simulink model "WaterTreatmentProcess"  (R2015b)
settings: Solver=VariableStepAuto  StartTime=0.0  StopTime=10.0  RelTol=1e-3
model workspace (MAT data in the model file):
  C0 = 1
  g = 9.81
  height = 1
  lenght = 12
  width = 3
settings Model: Creator=aemili  LastModifiedBy=andrea.emili

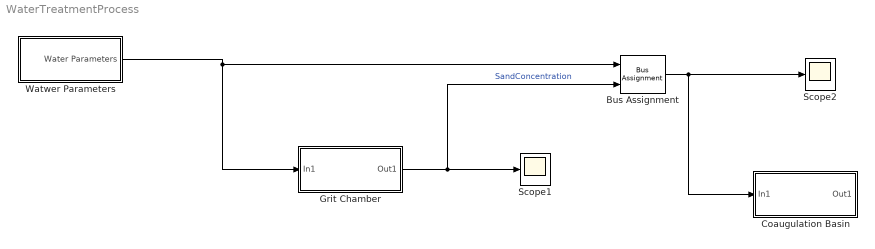
== system WaterTreatmentProcess ==
  Bus Assignment : BusAssignment  AssignedSignals=SandConcentration
  Coaugulation Basin : Subsystem
  Grit Chamber : Subsystem
  Scope1 : Scope
  Scope2 : Scope
  Watwer Parameters : Subsystem
  wires:
  Watwer Parameters/1(Water Parameters) -> Bus Assignment/1, Grit Chamber/1(In1)
  Grit Chamber/1(Out1) -> Bus Assignment/2, Scope1/1  "SandConcentration"
  Bus Assignment/1 -> Coaugulation Basin/1(In1), Scope2/1

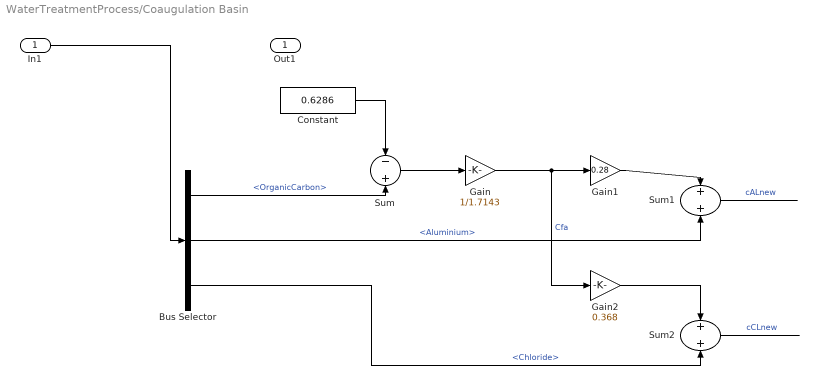
== system WaterTreatmentProcess/Coaugulation Basin ==
  In1 : Inport
  Bus Selector : BusSelector  OutputSignals=OrganicCarbon,Aluminium,Chloride
  Constant : Constant  Value=0.6286
  Gain : Gain  Gain=1/1.7143
  Gain1 : Gain  Gain=0.28
  Gain2 : Gain  Gain=0.368
  Sum : Sum  Inputs=-|+
  Sum1 : Sum  Inputs=+|+
  Sum2 : Sum  Inputs=+|+
  Out1 : Outport
  wires:
  In1/1 -> Bus Selector/1
  Sum/1 -> Gain/1
  Gain/1 -> Gain2/1, Gain1/1  "Cfa"
  Bus Selector/2 -> Sum1/2  "<Aluminium>"
  Bus Selector/3 -> Sum2/2  "<Chloride>"
  Gain1/1 -> Sum1/1
  Bus Selector/1 -> Sum/2  "<OrganicCarbon>"
  Constant/1 -> Sum/1
  Gain2/1 -> Sum2/1
  Sum2/1 -> ?  "cCLnew"
  Sum1/1 -> ?  "cALnew"

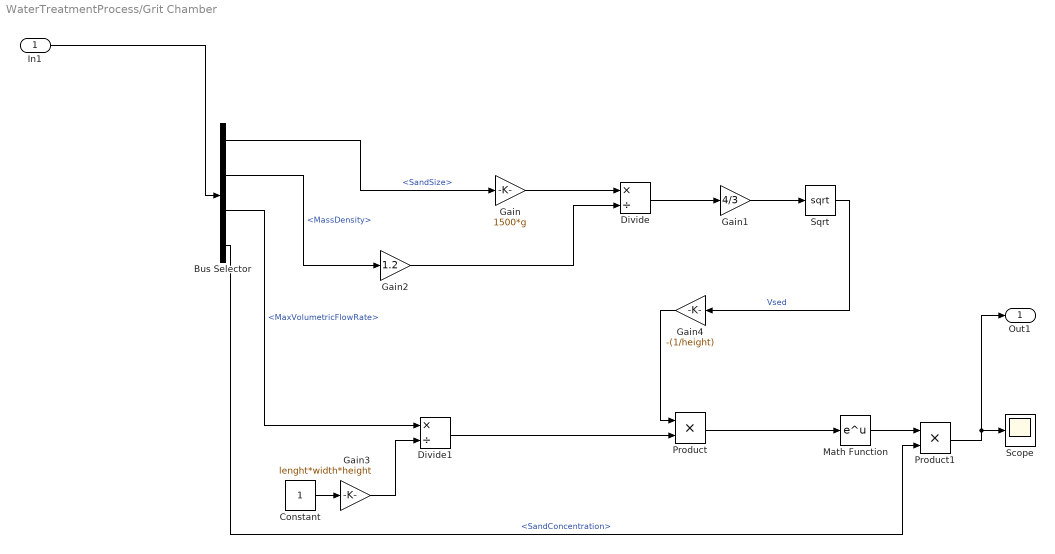
== system WaterTreatmentProcess/Grit Chamber ==
  In1 : Inport
  Bus Selector : BusSelector  OutputSignals=SandSize,MassDensity,MaxVolumetricFlowRate,SandConcentration
  Constant : Constant
  Divide : Product  Inputs=*/
  Divide1 : Product  Inputs=*/
  Gain : Gain  Gain=1500*g
  Gain1 : Gain  Gain=4/3
  Gain2 : Gain  Gain=1.2
  Gain3 : Gain  Gain=lenght*width*height
  Gain4 : Gain  Gain=-(1/height)
  Math Function : Math  SaturateOnIntegerOverflow=on
  Product : Product
  Product1 : Product
  Scope : Scope
  Sqrt : Sqrt  SaturateOnIntegerOverflow=on
  Out1 : Outport
  wires:
  In1/1 -> Bus Selector/1
  Bus Selector/1 -> Gain/1  "<SandSize>"
  Gain/1 -> Divide/1
  Bus Selector/2 -> Gain2/1  "<MassDensity>"
  Gain2/1 -> Divide/2
  Divide/1 -> Gain1/1
  Gain1/1 -> Sqrt/1
  Bus Selector/3 -> Divide1/1  "<MaxVolumetricFlowRate>"
  Divide1/1 -> Product/2
  Sqrt/1 -> Gain4/1  "Vsed"
  Gain4/1 -> Product/1
  Product/1 -> Math Function/1
  Math Function/1 -> Product1/1
  Product1/1 -> Out1/1, Scope/1
  Constant/1 -> Gain3/1
  Gain3/1 -> Divide1/2
  Bus Selector/4 -> Product1/2  "<SandConcentration>"

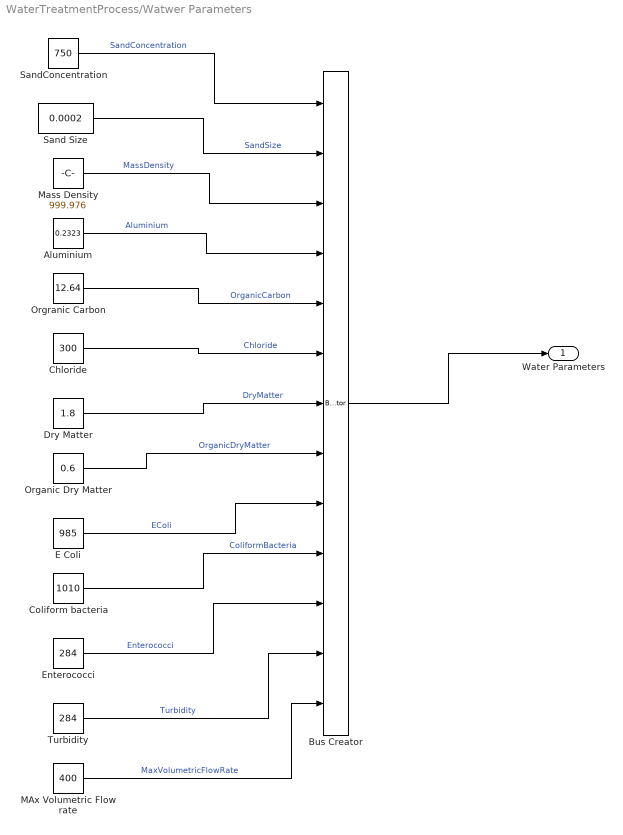
== system WaterTreatmentProcess/Watwer Parameters ==
  "Aluminium " : Constant  Value=0.2323
  Bus Creator : BusCreator  Inputs='SandConcentration','SandSize','MassDensity','Aluminium','OrganicCarbon','Chloride','DryMatter','OrganicDryMatter','EColi','ColiformBacteria','Enterococci','Turbidity','MaxVolumetricFlowRate'
  Chloride : Constant  Value=300
  Coliform bacteria : Constant  Value=1010
  Dry Matter : Constant  Value=1.8
  "E Coli " : Constant  Value=985
  "Enterococci " : Constant  Value=284
  MAx Volumetric Flow rate : Constant  Value=400
  Mass Density : Constant  Value=999.976
  Organic Dry Matter : Constant  Value=0.6
  "Orgranic Carbon " : Constant  Value=12.64
  Sand Size : Constant  Value=0.0002
  SandConcentration : Constant  Value=750
  Turbidity : Constant  Value=284
  Water Parameters : Outport
  wires:
  Bus Creator/1 -> Water Parameters/1
  SandConcentration/1 -> Bus Creator/1  "SandConcentration"
  Sand Size/1 -> Bus Creator/2  "SandSize"
  Mass Density/1 -> Bus Creator/3  "MassDensity"
  "Aluminium "/1 -> Bus Creator/4  "Aluminium"
  "Orgranic Carbon "/1 -> Bus Creator/5  "OrganicCarbon"
  Chloride/1 -> Bus Creator/6  "Chloride"
  Dry Matter/1 -> Bus Creator/7  "DryMatter"
  Organic Dry Matter/1 -> Bus Creator/8  "OrganicDryMatter"
  "E Coli "/1 -> Bus Creator/9  "EColi"
  Coliform bacteria/1 -> Bus Creator/10  "ColiformBacteria"
  "Enterococci "/1 -> Bus Creator/11  "Enterococci"
  Turbidity/1 -> Bus Creator/12  "Turbidity"
  MAx Volumetric Flow rate/1 -> Bus Creator/13  "MaxVolumetricFlowRate"
